simulink model "Final"  (R2018b)
settings: Solver=FixedStepAuto  StartTime=0.0  StopTime=1  RelTol=1e-3  EnableMultiTasking=on
values from neighbouring files (symbols this model uses):
  A = [-(bm*(n^2) + bg)/(Jm*(n^2) + Jg) Kt*n/(Jm*(n^2) + Jg) ... (first row only)    [DC_motor_geared_integral_discrete_sysid23.m]    (also in DC_motor_geared_lqr_discrete_sysid23.m; finalScript.m; finalScriptV2.m; precompensatorVSintegrator.m)
  B = [0 ... (first row only)    [DC_motor_geared_integral_discrete_sysid23.m]    (also in DC_motor_geared_lqr_discrete_sysid23.m; finalScript.m; finalScriptV2.m; precompensatorVSintegrator.m)
  C = [1 0]    [DC_motor_geared_integral_discrete_sysid23.m]    (also in DC_motor_geared_lqr_discrete_sysid23.m = eye(2); finalScript.m; finalScriptV2.m; precompensatorVSintegrator.m = eye(2))
  D = [0]    [DC_motor_geared_integral_discrete_sysid23.m]    (also in DC_motor_geared_lqr_discrete_sysid23.m = [0;0]; finalScript.m; finalScriptV2.m; precompensatorVSintegrator.m)
  Kdi = dlqr(Ad,Bd,Q,R)    [finalScript.m]    (also in finalScriptV2.m)
  n = 16.5    [DC_motor_geared_integral_discrete_sysid23.m]    (also in DC_motor_geared_lqr_discrete_sysid23.m; finalScript.m; finalScriptV2.m)
  Tsc = 1/20000    (= 5e-05)    [DC_motor_geared_integral_discrete_sysid23.m]    (also in DC_motor_geared_lqr_discrete_sysid23.m = 1e-05; finalScript.m; finalScriptV2.m = 0.001)
undefined symbols (not defined in the file or in its folder): DiscIntNeverNeededParam
libraries: dspswit3 x29, simulink x10, powerlib_meascontrol x4, dspsigops x4, pePwmGenerator x4, peLuenbergerObserver x2, peGeneralControl x1
settings Model: Creator=Roberto  LastModifiedBy=Roberto
settings SolverCC: AutoInsertRateTranBlk=on
settings OptimizationCC: EnhancedBackFolding=on  PassReuseOutputArgsAs=Individual arguments  MaxStackSize=64  OptimizeBlockOrder=speed  DifferentSizesBufferReuse=on  OptimizationCustomize=off
settings DebuggingCC: ParameterTunabilityLossMsg=error
settings HardwareCC: ProdBitPerPointer=32  ProdBitPerSizeT=32  ProdBitPerPtrDiffT=32  ProdLargestAtomicInteger=Long  ProdLargestAtomicFloat=Double  ProdWordSize=32  ProdHWDeviceType=ARM Compatible->ARM Cortex
settings SFSimCC: MATLABDynamicMemAlloc=off
settings RTWCC: SystemTargetFile=ert.tlc  HardwareBoard=STM32F746G-Discovery  TemplateMakefile=ert_default_tmf  GenerateReport=on  Toolchain=GNU Tools for ARM Embedded Processors  IncludeHyperlinkInReport=on  LaunchReport=on  GenerateTraceInfo=on  GenerateTraceReport=on  GenerateTraceReportSl=on  GenerateTraceReportSf=on  GenerateTraceReportEml=on
settings CodeAppCC: ForceParamTrailComments=on  IgnoreCustomStorageClasses=off  OperatorAnnotations=on  SimulinkDataObjDesc=on  SFDataObjDesc=on  InsertBlockDesc=on

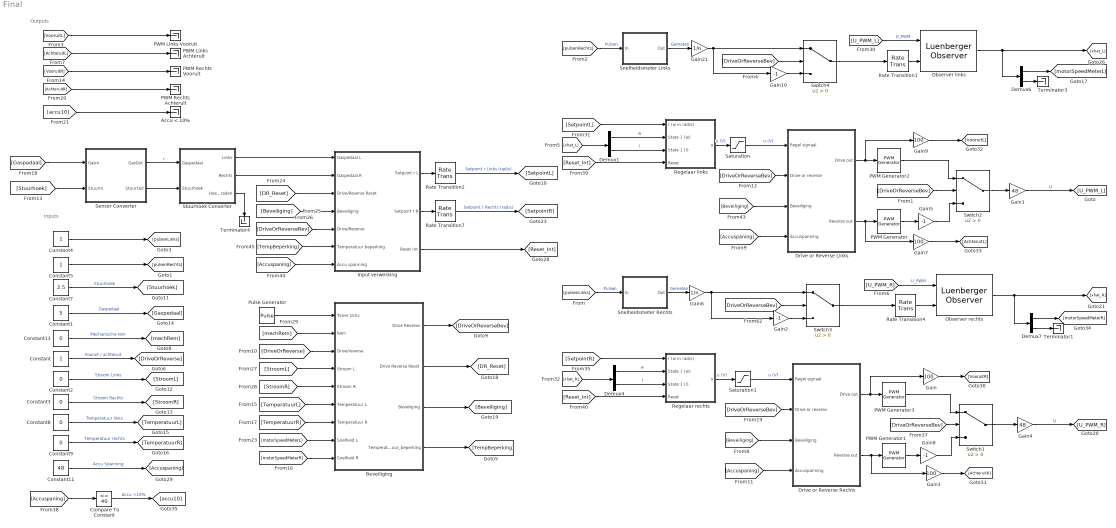
== system Final ==
  note: Inputs
  note: Outputs
  Accu < 10% : Terminator
  Beveiliging : Subsystem
  Compare To Constant : simulink/Logic and Bit Operations/Compare To Constant  relop=<=  const=40  OutDataTypeStr=boolean
  Constant : Constant
  Constant1 : Constant  Value=5
  Constant11 : Constant  Value=48
  Constant{2..3,8..9,13} (5 alike) : Constant  Value=0
  Constant4 : Constant
  Constant5 : Constant
  Constant7 : Constant  Value=2.5
  Demux{1,4,6..7} (4 alike) : Demux  Outputs=2
  Drive or Reverse Links : Subsystem
  Drive or Reverse Rechts : Subsystem
  Gain{,3,7,9} (4 alike) : Gain  Gain=100
  Gain1 : Gain  Gain=48
  Gain{2,5,8,10} (4 alike) : Gain  Gain=-1
  Gain21 : Gain  Gain=1/n
  Gain4 : Gain  Gain=48
  Gain6 : Gain  Gain=1/n
  Input verwerking : Subsystem
  Observer links : peLuenbergerObserver/Luenberger Observer  StateSpaceType=Continuous-time  Ad=Adh  Bd=Bdh  Cd=C  Dd=0  A=A  B=B  C=C  D=D  ObserverDesign=Observer gain  Ld=L  DesiredEigenvalues=eigenVal  x0=[0 0]  Tsd=0.1  Ts=1e-6
  Observer rechts : peLuenbergerObserver/Luenberger Observer  StateSpaceType=Continuous-time  Ad=Adh  Bd=Bdh  Cd=C  Dd=0  A=A  B=B  C=C  D=D  ObserverDesign=Observer gain  Ld=L  DesiredEigenvalues=eigenVal  x0=[0 0]  Tsd=0.1  Ts=1e-6
  PWM Generator{,1..3} (4 alike) : pePwmGenerator/PWM Generator  CarrCount=Up  Tper=1/20000  Ts=1e-6
  PWM Links Achteruit : Terminator
  PWM Links Vooruit : Terminator
  PWM Rechts Achteruit : Terminator
  PWM Rechts Vooruit : Terminator
  Pulse Generator : DiscretePulseGenerator  SampleTime=1/2000
  Rate Transition1 : RateTransition  OutPortSampleTime=1e-6
  Rate Transition2 : RateTransition  OutPortSampleTime=Tsc
  Rate Transition4 : RateTransition  OutPortSampleTime=1e-6
  Rate Transition7 : RateTransition  OutPortSampleTime=Tsc
  Regelaar links : Subsystem
  Regelaar rechts : Subsystem
  Saturation : Saturate  UpperLimit=60  LowerLimit=-60
  Saturation1 : Saturate  UpperLimit=60  LowerLimit=-60
  Sensor Converter : Subsystem
  Snelheidsmeter Links : Subsystem
  Snelheidsmeter Rechts : Subsystem
  Stuurhoek Converter : Subsystem
  Switch{1..4} (4 alike) : Switch  Criteria=u2 > Threshold
  Terminator1 : Terminator
  Terminator3 : Terminator
  Terminator4 : Terminator
  wires:
  Gain1/1 -> [U_PWM_L]  "U"
  Switch2/1 -> Gain1/1
  Demux1/2 -> Regelaar links/3(State 1 (I))  "I"
  Demux1/1 -> Regelaar links/2(State 1 (w))  "w"
  [Reset_Int] -> Regelaar links/4(Reset)
  [xhat_L] -> Demux1/1
  [U_PWM_L] -> Observer links/1  "U_PWM"
  [pulsenRechts] -> Snelheidsmeter Links/1(In)  "Pulsen"
  Rate Transition1/1 -> Observer links/2
  Snelheidsmeter Links/1(Out) -> Gain21/1  "Gemeten"
  Switch4/1 -> Rate Transition1/1
  Observer links/1 -> Demux6/1, [xhat_L]
  Beveiliging/1("Drive Reverse ") -> [DriveOrReverseBev]
  [Gaspedaal] -> Sensor Converter/1(GasIn)
  Stuurhoek Converter/1(Links) -> Input verwerking/1(Gaspedaal L)
  Input verwerking/1(Setpoint r L) -> Rate Transition2/1
  [Stuurhoek] -> Sensor Converter/2(StuurIn)
  Input verwerking/3(Reset Int) -> [Reset_Int]
  Sensor Converter/2(StuurOut) -> Stuurhoek Converter/2(Stuurhoek)
  [DriveOrReverse] -> Beveiliging/3(Drive/reverse)
  [motorSpeedMeterR] -> Beveiliging/9(Snelheid R)
  [TemperatuurL] -> Beveiliging/6(Temperatuur L)
  [StroomR] -> Beveiliging/5(Stroom R)
  [StroomL] -> Beveiliging/4(Stroom L)
  Beveiliging/3(Beveiliging) -> [Beveiliging]
  [motorSpeedMeterL] -> Beveiliging/8(Snelheid L)
  Input verwerking/2(Setpoint r R) -> Rate Transition7/1
  Beveiliging/2(Drive Reverse Reset) -> [DR_Reset]
  Stuurhoek Converter/2(Rechts) -> Input verwerking/2(Gaspedaal R)
  [mechRem] -> Beveiliging/2(Rem)
  [DR_Reset] -> Input verwerking/3(Drive/Reverse Reset)
  [Beveiliging] -> Input verwerking/4(Beveiliging)
  Pulse Generator/1 -> Beveiliging/1(Timer 1khz)
  [DriveOrReverseBev] -> Input verwerking/5(Drive/Reverse)
  Rate Transition7/1 -> [SetpointR]  "Setpoint r Rechts (rad/s)"
  Rate Transition2/1 -> [SetpointL]  "Setpoint r Links (rad/s)"
  [TemperatuurR] -> Beveiliging/7(Temperatuur R)
  Observer rechts/1 -> Demux7/1, [xhat_R]
  Demux4/2 -> Regelaar rechts/3(State 1 (I))  "I"
  Rate Transition4/1 -> Observer rechts/2
  Switch1/1 -> Gain4/1
  [U_PWM_R] -> Observer rechts/1  "U_PWM"
  Snelheidsmeter Rechts/1(Out) -> Gain6/1  "Gemeten"
  [Reset_Int] -> Regelaar rechts/4(Reset)
  [xhat_R] -> Demux4/1
  [pulsenLinks] -> Snelheidsmeter Rechts/1(In)  "Pulsen"
  Demux4/1 -> Regelaar rechts/2(State 1 (w))  "w"
  Gain4/1 -> [U_PWM_R]  "U"
  [SetpointL] -> Regelaar links/1(r (w in rad/s))
  [SetpointR] -> Regelaar rechts/1(r (w in rad/s))
  [Beveiliging] -> Drive or Reverse Rechts/3(Beveiliging)
  [DriveOrReverseBev] -> Switch1/2
  Drive or Reverse Rechts/1(Drive out) -> Gain/1, PWM Generator3/1
  [Accuspaning] -> Drive or Reverse Rechts/4(Accuspanning)
  [DriveOrReverseBev] -> Drive or Reverse Rechts/2(Drive or reverse)
  Drive or Reverse Rechts/2(Reverse out) -> Gain3/1, PWM Generator1/1
  Regelaar rechts/1(u) -> Saturation1/1  "u (V)"
  [Beveiliging] -> Drive or Reverse Links/3(Beveiliging)
  [DriveOrReverseBev] -> Switch2/2
  Drive or Reverse Links/1(Drive out) -> Gain9/1, PWM Generator2/1
  [Accuspaning] -> Drive or Reverse Links/4(Accuspanning)
  [DriveOrReverseBev] -> Drive or Reverse Links/2(Drive or reverse)
  Drive or Reverse Links/2(Reverse out) -> Gain7/1, PWM Generator/1
  Regelaar links/1(u) -> Saturation/1  "u (V)"
  Constant1/1 -> [Gaspedaal]  "Gaspedaal"
  Constant13/1 -> [mechRem]  "Mechanische rem"
  Constant/1 -> [DriveOrReverse]  "Vooruit / achteruit"
  Constant2/1 -> [StroomL]  "Stroom Links"
  Constant9/1 -> [TemperatuurR]  "Temperatuur rechts"
  Constant7/1 -> [Stuurhoek]  "Stuurhoek"
  Constant3/1 -> [StroomR]  "Stroom Rechts"
  Constant8/1 -> [TemperatuurL]  "Temperatuur links"
  Constant11/1 -> [Accuspaning]  "Accu Spanning"
  Beveiliging/4(Temperatuur_beperking) -> [TempBeperking]
  [Accuspaning] -> Input verwerking/7(Accu spanning)
  [TempBeperking] -> Input verwerking/6(Temperatuur beperking)
  Gain6/1 -> Gain2/1, Switch3/1
  [DriveOrReverseBev] -> Switch3/2
  Gain2/1 -> Switch3/3
  Switch3/1 -> Rate Transition4/1
  Gain21/1 -> Gain10/1, Switch4/1
  Gain10/1 -> Switch4/3
  [DriveOrReverseBev] -> Switch4/2
  Gain5/1 -> Switch2/3
  Gain8/1 -> Switch1/3
  PWM Generator/1 -> Gain5/1
  PWM Generator2/1 -> Switch2/1
  PWM Generator1/1 -> Gain8/1
  PWM Generator3/1 -> Switch1/1
  Saturation/1 -> Drive or Reverse Links/1(Regel signaal)  "u (V)"
  Saturation1/1 -> Drive or Reverse Rechts/1(Regel signaal)  "u (V)"
  Demux6/1 -> [motorSpeedMeterL]
  Demux7/1 -> [motorSpeedMeterR]
  Demux7/2 -> Terminator1/1
  Demux6/2 -> Terminator3/1
  Compare To Constant/1 -> [accu10]  "Accu <10%"
  [Accuspaning] -> Compare To Constant/1
  Sensor Converter/1(GasOut) -> Stuurhoek Converter/1("Gaspedaal ")  "r"
  Stuurhoek Converter/3(Hoek in graden) -> Terminator4/1
  Constant4/1 -> [pulsenLinks]
  Constant5/1 -> [pulsenRechts]
  Gain/1 -> [VooruitR]
  Gain3/1 -> [AchteruitR]
  Gain7/1 -> [AchteruitL]
  Gain9/1 -> [VooruitL]
  [VooruitL] -> PWM Links Vooruit/1
  [AchteruitL] -> PWM Links Achteruit/1
  [VooruitR] -> PWM Rechts Vooruit/1
  [AchteruitR] -> PWM Rechts Achteruit/1
  [accu10] -> Accu < 10%/1

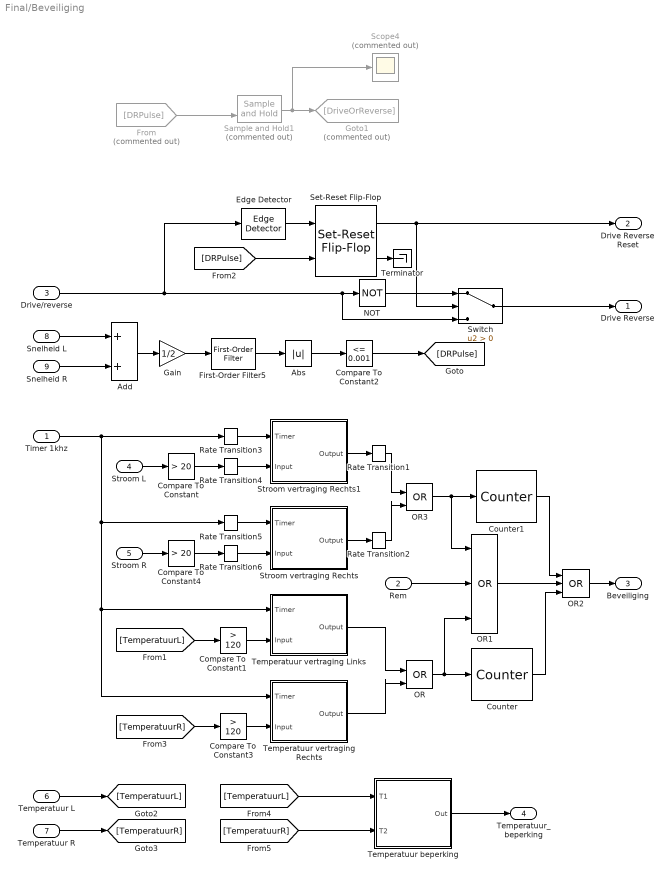
== system Final/Beveiliging ==
  Timer 1khz : Inport
  Rem : Inport  Port=2
  Drive/reverse : Inport  Port=3
  Stroom L : Inport  Port=4
  Stroom R : Inport  Port=5
  Temperatuur L : Inport  Port=6
  Temperatuur R : Inport  Port=7
  Snelheid L : Inport  Port=8
  Snelheid R : Inport  Port=9
  Abs : Abs
  Add : Sum
  Compare To Constant : simulink/Logic and Bit Operations/Compare To Constant  relop=>  const=20  OutDataTypeStr=boolean
  Compare To Constant1 : simulink/Logic and Bit Operations/Compare To Constant  relop=>  const=120  OutDataTypeStr=boolean
  Compare To Constant2 : simulink/Logic and Bit Operations/Compare To Constant  relop=<=  const=0.001  OutDataTypeStr=boolean
  Compare To Constant3 : simulink/Logic and Bit Operations/Compare To Constant  relop=>  const=120  OutDataTypeStr=boolean
  Compare To Constant4 : simulink/Logic and Bit Operations/Compare To Constant  relop=>  const=20  OutDataTypeStr=boolean
  Counter : dspswit3/Counter  Direction=Up  CountEvent=Rising edge  CounterSize=32 bits  MaxCount=255  InitialCount=0  Output=Hit  HitValue=3  ResetInput=off  SamplesPerFrame=1  Ts=1  CntDtype=double  HitDtype=Logical
  Counter1 : dspswit3/Counter  Direction=Up  CountEvent=Rising edge  CounterSize=32 bits  MaxCount=255  InitialCount=0  Output=Hit  HitValue=2  ResetInput=off  SamplesPerFrame=1  Ts=1  CntDtype=double  HitDtype=Logical
  Edge Detector : powerlib_meascontrol/Logic/Edge Detector  model=Either  ic=0  Ts=-1
      settings: SourceProductName=Simscape Power Systems  SourceProductBaseCode=PS
  First-Order Filter5 : powerlib_meascontrol/Filters/First-Order Filter  FilterType=Lowpass  Tc=10e-3  Ts=Tsc  Initialize=on  Vac_Init=[0, 0, 50]  Vdc_Init=0  PlotResponse=off  FreqRange="[0,  200,  1]"
      settings: SourceProductName=Simscape Power Systems
  From : From  Commented=on  GotoTag=DRPulse
  Gain : Gain  Gain=1/2
  Goto1 : Goto  Commented=on  GotoTag=DriveOrReverse
  NOT : Logic  Operator=NOT  IconShape=distinctive  AllPortsSameDT=off  OutDataTypeStr=boolean
  OR : Logic  Operator=OR  IconShape=distinctive  AllPortsSameDT=off  OutDataTypeStr=boolean
  OR1 : Logic  Operator=OR  Inputs=3  IconShape=distinctive  AllPortsSameDT=off  OutDataTypeStr=boolean
  OR2 : Logic  Operator=OR  Inputs=3  IconShape=distinctive  AllPortsSameDT=off  OutDataTypeStr=boolean
  OR3 : Logic  Operator=OR  IconShape=distinctive  AllPortsSameDT=off  OutDataTypeStr=boolean
  Rate Transition{1..6} (6 alike) : RateTransition
  Sample and Hold1 : powerlib_meascontrol/Additional Components/Sample and Hold  Commented=on  ic=0  Ts=0
      settings: SourceProductName=Simscape Power Systems  SourceProductBaseCode=PS
  Scope4 : Scope  Commented=on
  Set-Reset Flip-Flop : peGeneralControl/Set-Reset Flip-Flop  LabelModeActiveChoice=Discrete  UndefState=Set  Q0=0  Ts=-1
  Stroom vertraging Rechts : Subsystem
  Stroom vertraging Rechts1 : Subsystem
  Switch : Switch  Criteria=u2 > Threshold
  Temperatuur beperking : Subsystem
  Temperatuur vertraging Links : Subsystem
  "Temperatuur vertraging Rechts " : Subsystem
  Terminator : Terminator
  "Drive Reverse " : Outport
  Drive Reverse Reset : Outport  Port=2
  Beveiliging : Outport  Port=3
  Temperatuur_beperking : Outport  Port=4
  wires:
  Stroom L/1 -> Compare To Constant/1
  Compare To Constant1/1 -> Temperatuur vertraging Links/2(Input)
  Edge Detector/1 -> Set-Reset Flip-Flop/1
  Set-Reset Flip-Flop/1 -> Switch/2, Drive Reverse Reset/1
  Sample and Hold1/1 -> Scope4/1, Goto1/1
  Abs/1 -> Compare To Constant2/1
  Compare To Constant2/1 -> [DRPulse]
  [DRPulse] -> Set-Reset Flip-Flop/2
  Drive/reverse/1 -> Edge Detector/1, Switch/3, NOT/1
  From/1 -> Sample and Hold1/2
  Snelheid L/1 -> Add/1
  Snelheid R/1 -> Add/2
  Add/1 -> Gain/1
  Gain/1 -> First-Order Filter5/1
  Compare To Constant3/1 -> "Temperatuur vertraging Rechts "/2(Input)
  Timer 1khz/1 -> Rate Transition3/1, Rate Transition5/1, Temperatuur vertraging Links/1(Timer), "Temperatuur vertraging Rechts "/1(Timer)
  Compare To Constant4/1 -> Rate Transition6/1
  Stroom R/1 -> Compare To Constant4/1
  Rem/1 -> OR1/2
  Switch/1 -> "Drive Reverse "/1
  NOT/1 -> Switch/1
  OR/1 -> OR1/3, Counter/1
  Temperatuur vertraging Links/1(Output) -> OR/1
  "Temperatuur vertraging Rechts "/1(Output) -> OR/2
  OR2/1 -> Beveiliging/1
  Counter/1 -> OR2/3
  OR1/1 -> OR2/2
  Set-Reset Flip-Flop/2 -> Terminator/1
  First-Order Filter5/1 -> Abs/1
  Temperatuur L/1 -> [TemperatuurL]
  Temperatuur R/1 -> [TemperatuurR]
  [TemperatuurL] -> Compare To Constant1/1
  [TemperatuurR] -> Compare To Constant3/1
  [TemperatuurL] -> Temperatuur beperking/1(T1)
  [TemperatuurR] -> Temperatuur beperking/2(T2)
  Temperatuur beperking/1(Out) -> Temperatuur_beperking/1
  Compare To Constant/1 -> Rate Transition4/1
  Stroom vertraging Rechts1/1(Output) -> Rate Transition1/1
  Stroom vertraging Rechts/1(Output) -> Rate Transition2/1
  OR3/1 -> Counter1/1, OR1/1
  Counter1/1 -> OR2/1
  Rate Transition6/1 -> Stroom vertraging Rechts/2(Input)
  Rate Transition5/1 -> Stroom vertraging Rechts/1(Timer)
  Rate Transition4/1 -> Stroom vertraging Rechts1/2(Input)
  Rate Transition3/1 -> Stroom vertraging Rechts1/1(Timer)
  Rate Transition2/1 -> OR3/2
  Rate Transition1/1 -> OR3/1

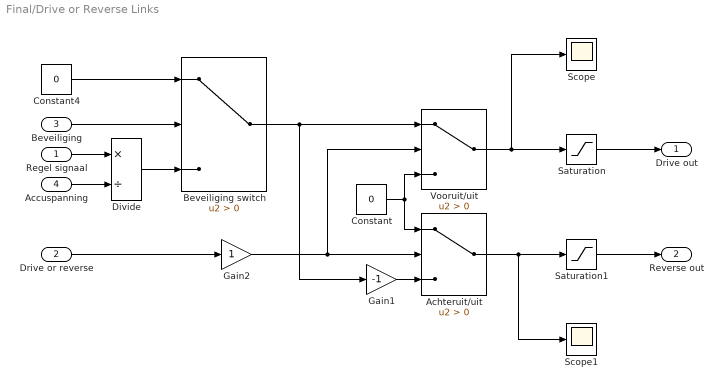
== system Final/Drive or Reverse Links ==
  Regel signaal : Inport
  Drive or reverse : Inport  Port=2
  Beveiliging : Inport  Port=3
  Accuspanning : Inport  Port=4
  Achteruit/uit : Switch  Criteria=u2 > Threshold
  Beveiliging switch : Switch  Criteria=u2 > Threshold
  Constant : Constant  Value=0
  Constant4 : Constant  Value=0
  Divide : Product  Inputs=*/
  Gain1 : Gain  Gain=-1
  Gain2 : Gain
  Saturation : Saturate  UpperLimit=1  LowerLimit=0
  Saturation1 : Saturate  UpperLimit=1  LowerLimit=0
  Scope : Scope
  Scope1 : Scope
  Vooruit/uit : Switch  Criteria=u2 > Threshold
  Drive out : Outport
  Reverse out : Outport  Port=2
  wires:
  Gain1/1 -> Achteruit/uit/3
  Constant4/1 -> Beveiliging switch/1
  Constant/1 -> Achteruit/uit/1, Vooruit/uit/3
  Beveiliging switch/1 -> Gain1/1, Vooruit/uit/1
  Beveiliging/1 -> Beveiliging switch/2
  Achteruit/uit/1 -> Saturation1/1, Scope1/1
  Gain2/1 -> Vooruit/uit/2, Achteruit/uit/2
  Drive or reverse/1 -> Gain2/1
  Vooruit/uit/1 -> Saturation/1, Scope/1
  Accuspanning/1 -> Divide/2
  Divide/1 -> Beveiliging switch/3
  Regel signaal/1 -> Divide/1
  Saturation/1 -> Drive out/1
  Saturation1/1 -> Reverse out/1

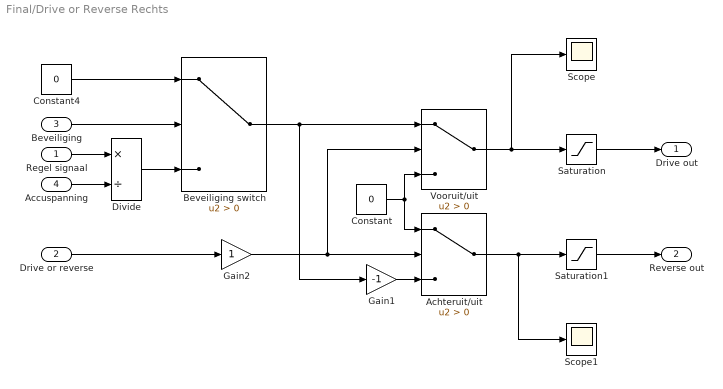
== system Final/Drive or Reverse Rechts ==
  Regel signaal : Inport
  Drive or reverse : Inport  Port=2
  Beveiliging : Inport  Port=3
  Accuspanning : Inport  Port=4
  Achteruit/uit : Switch  Criteria=u2 > Threshold
  Beveiliging switch : Switch  Criteria=u2 > Threshold
  Constant : Constant  Value=0
  Constant4 : Constant  Value=0
  Divide : Product  Inputs=*/
  Gain1 : Gain  Gain=-1
  Gain2 : Gain
  Saturation : Saturate  UpperLimit=1  LowerLimit=0
  Saturation1 : Saturate  UpperLimit=1  LowerLimit=0
  Scope : Scope
  Scope1 : Scope
  Vooruit/uit : Switch  Criteria=u2 > Threshold
  Drive out : Outport
  Reverse out : Outport  Port=2
  wires:
  Gain1/1 -> Achteruit/uit/3
  Constant4/1 -> Beveiliging switch/1
  Constant/1 -> Achteruit/uit/1, Vooruit/uit/3
  Beveiliging switch/1 -> Gain1/1, Vooruit/uit/1
  Beveiliging/1 -> Beveiliging switch/2
  Achteruit/uit/1 -> Saturation1/1, Scope1/1
  Gain2/1 -> Vooruit/uit/2, Achteruit/uit/2
  Drive or reverse/1 -> Gain2/1
  Vooruit/uit/1 -> Saturation/1, Scope/1
  Accuspanning/1 -> Divide/2
  Divide/1 -> Beveiliging switch/3
  Regel signaal/1 -> Divide/1
  Saturation/1 -> Drive out/1
  Saturation1/1 -> Reverse out/1

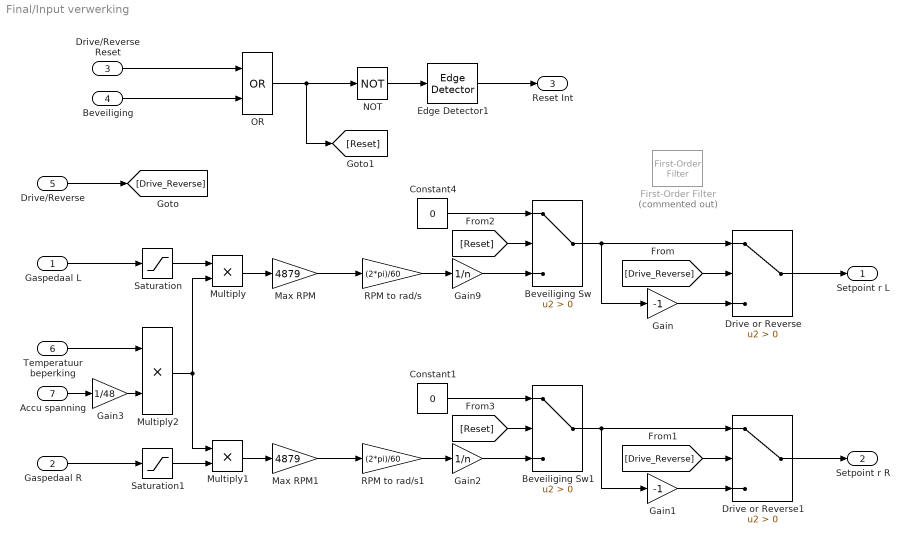
== system Final/Input verwerking ==
  Gaspedaal L : Inport
  Gaspedaal R : Inport  Port=2
  Drive/Reverse Reset : Inport  Port=3
  Beveiliging : Inport  Port=4
  Drive/Reverse : Inport  Port=5
  Temperatuur beperking : Inport  Port=6
  Accu spanning : Inport  Port=7
  Beveiliging Sw : Switch  Criteria=u2 > Threshold
  Beveiliging Sw1 : Switch  Criteria=u2 > Threshold
  Constant1 : Constant  Value=0
  Constant4 : Constant  Value=0
  Drive or Reverse : Switch  Criteria=u2 > Threshold
  Drive or Reverse1 : Switch  Criteria=u2 > Threshold
  Edge Detector1 : dspswit3/Edge Detector  InputProcessing=Columns as channels (frame based)
      settings: SourceProductName=DSP System Toolbox  SourceProductBaseCode=DS
  First-Order Filter : powerlib_meascontrol/Filters/First-Order Filter  Commented=on  FilterType=Lowpass  Tc=10e-2  Ts=0  Initialize=on  Vac_Init=[0, 0, 60]  Vdc_Init=0  PlotResponse=off  FreqRange="[0,  200,  1]"
      settings: SourceProductName=Simscape Power Systems
  Gain : Gain  Gain=-1
  Gain1 : Gain  Gain=-1
  Gain2 : Gain  Gain=1/n
  Gain3 : Gain  Gain=1/48
  Gain9 : Gain  Gain=1/n
  Max RPM : Gain  Gain=4879
  Max RPM1 : Gain  Gain=4879
  Multiply : Product
  Multiply1 : Product
  Multiply2 : Product
  NOT : Logic  Operator=NOT  IconShape=distinctive  AllPortsSameDT=off  OutDataTypeStr=boolean
  OR : Logic  Operator=OR  IconShape=distinctive  AllPortsSameDT=off  OutDataTypeStr=boolean
  RPM to rad/s : Gain  Gain=(2*pi)/60
  RPM to rad/s1 : Gain  Gain=(2*pi)/60
  Saturation : Saturate  UpperLimit=1  LowerLimit=0
  Saturation1 : Saturate  UpperLimit=1  LowerLimit=0
  Setpoint r L : Outport
  Setpoint r R : Outport  Port=2
  Reset Int : Outport  Port=3
  wires:
  Constant4/1 -> Beveiliging Sw/1
  Max RPM/1 -> RPM to rad/s/1
  RPM to rad/s/1 -> Gain9/1
  Gaspedaal L/1 -> Saturation/1
  OR/1 -> [Reset], NOT/1
  Gain9/1 -> Beveiliging Sw/3
  Beveiliging Sw/1 -> Gain/1, Drive or Reverse/1
  Gain/1 -> Drive or Reverse/3
  [Drive_Reverse] -> Drive or Reverse/2
  Drive or Reverse/1 -> Setpoint r L/1
  Edge Detector1/1 -> Reset Int/1
  NOT/1 -> Edge Detector1/1
  Beveiliging/1 -> OR/2
  Drive/Reverse Reset/1 -> OR/1
  Max RPM1/1 -> RPM to rad/s1/1
  RPM to rad/s1/1 -> Gain2/1
  Drive or Reverse1/1 -> Setpoint r R/1
  Gaspedaal R/1 -> Saturation1/1
  Gain1/1 -> Drive or Reverse1/3
  Beveiliging Sw1/1 -> Gain1/1, Drive or Reverse1/1
  Constant1/1 -> Beveiliging Sw1/1
  [Drive_Reverse] -> Drive or Reverse1/2
  Gain2/1 -> Beveiliging Sw1/3
  Drive/Reverse/1 -> [Drive_Reverse]
  [Reset] -> Beveiliging Sw/2
  [Reset] -> Beveiliging Sw1/2
  Multiply/1 -> Max RPM/1
  Multiply1/1 -> Max RPM1/1
  Saturation1/1 -> Multiply1/2
  Saturation/1 -> Multiply/1
  Multiply2/1 -> Multiply/2, Multiply1/1
  Temperatuur beperking/1 -> Multiply2/1
  Accu spanning/1 -> Gain3/1
  Gain3/1 -> Multiply2/2

== system Final/Regelaar links ==
  r (w in rad/s) : Inport
  State 1 (w) : Inport  Port=2
  State 1 (I) : Inport  Port=3
  Reset : Inport  Port=4
  Discrete-Time Integrator2 : DiscreteIntegrator  gainval=1  ExternalReset=rising  SampleTime=Tsc  ICPrevOutput=DiscIntNeverNeededParam  ICPrevScaledInput=DiscIntNeverNeededParam
  Gain1 : Gain  Gain=Kdi(1:2)  Multiplication=Matrix(K*u)
  Gain4 : Gain  Gain=Kdi(3)
  Mux : Mux  Inputs=2
  Sum1 : Sum  Inputs=|+-
  Sum4 : Sum  Inputs=|+-
  u : Outport
  wires:
  r (w in rad/s)/1 -> Sum1/1
  State 1 (I)/1 -> Mux/2
  Mux/1 -> Gain1/1
  Gain1/1 -> Sum4/2
  Gain4/1 -> Sum4/1
  Sum4/1 -> u/1
  State 1 (w)/1 -> Mux/1, Sum1/2
  Sum1/1 -> Discrete-Time Integrator2/1
  Discrete-Time Integrator2/1 -> Gain4/1
  Reset/1 -> Discrete-Time Integrator2/2

== system Final/Regelaar rechts ==
  r (w in rad/s) : Inport
  State 1 (w) : Inport  Port=2
  State 1 (I) : Inport  Port=3
  Reset : Inport  Port=4
  Discrete-Time Integrator2 : DiscreteIntegrator  gainval=1  ExternalReset=rising  SampleTime=Tsc  ICPrevOutput=DiscIntNeverNeededParam  ICPrevScaledInput=DiscIntNeverNeededParam
  Gain1 : Gain  Gain=Kdi(1:2)  Multiplication=Matrix(K*u)
  Gain4 : Gain  Gain=Kdi(3)
  Mux : Mux  Inputs=2
  Sum1 : Sum  Inputs=|+-
  Sum4 : Sum  Inputs=|+-
  u : Outport
  wires:
  r (w in rad/s)/1 -> Sum1/1
  State 1 (I)/1 -> Mux/2
  Mux/1 -> Gain1/1
  Gain1/1 -> Sum4/2
  Gain4/1 -> Sum4/1
  Sum4/1 -> u/1
  State 1 (w)/1 -> Mux/1, Sum1/2
  Sum1/1 -> Discrete-Time Integrator2/1
  Discrete-Time Integrator2/1 -> Gain4/1
  Reset/1 -> Discrete-Time Integrator2/2

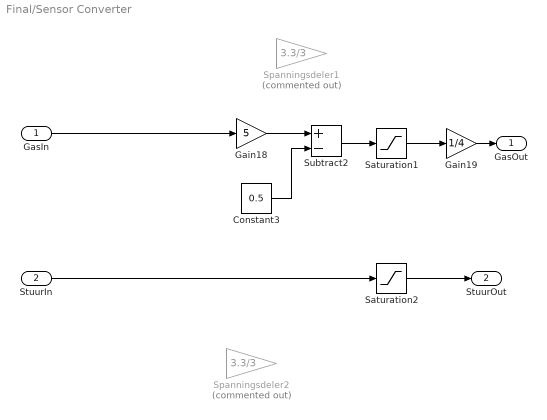
== system Final/Sensor Converter ==
  GasIn : Inport
  StuurIn : Inport  Port=2
  Constant3 : Constant  Value=0.5
  Gain18 : Gain  Gain=5
  Gain19 : Gain  Gain=1/4
  Saturation1 : Saturate  UpperLimit=4  LowerLimit=0
  Saturation2 : Saturate  UpperLimit=1  LowerLimit=0
  Spanningsdeler1 : Gain  Commented=on  Gain=3.3/3
  Spanningsdeler2 : Gain  Commented=on  Gain=3.3/3
  Subtract2 : Sum  Inputs=+-
  GasOut : Outport
  StuurOut : Outport  Port=2
  wires:
  Constant3/1 -> Subtract2/2
  Saturation1/1 -> Gain19/1
  GasIn/1 -> Gain18/1
  Gain18/1 -> Subtract2/1
  Gain19/1 -> GasOut/1
  Subtract2/1 -> Saturation1/1
  Saturation2/1 -> StuurOut/1
  StuurIn/1 -> Saturation2/1

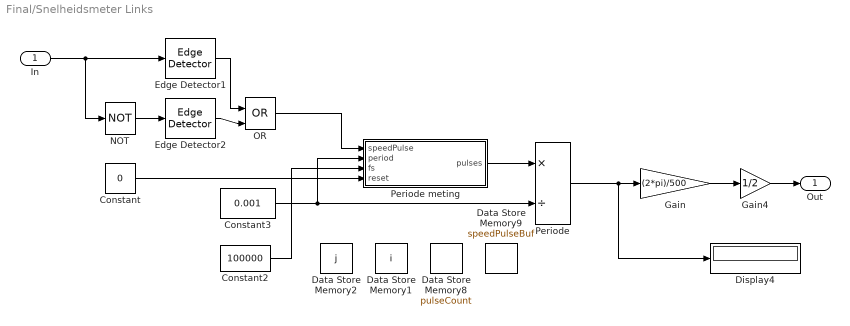
== system Final/Snelheidsmeter Links ==
  In : Inport
  Constant : Constant  Value=0
  Constant2 : Constant  Value=100000
  Constant3 : Constant  Value=0.001
  Data Store Memory1 : DataStoreMemory  DataStoreName=i  ReadBeforeWriteMsg=warning  WriteAfterWriteMsg=warning  WriteAfterReadMsg=warning  InitialValue=1  ShowAdditionalParam=off  OutDataTypeStr=uint32
  Data Store Memory2 : DataStoreMemory  DataStoreName=j  ReadBeforeWriteMsg=warning  WriteAfterWriteMsg=warning  WriteAfterReadMsg=warning  InitialValue=2  ShowAdditionalParam=off  OutDataTypeStr=uint32
  Data Store Memory8 : DataStoreMemory  DataStoreName=pulseCount  ReadBeforeWriteMsg=warning  WriteAfterWriteMsg=warning  WriteAfterReadMsg=warning  ShowAdditionalParam=off  OutDataTypeStr=uint32
  Data Store Memory9 : DataStoreMemory  DataStoreName=speedPulseBuf  ReadBeforeWriteMsg=warning  WriteAfterWriteMsg=warning  WriteAfterReadMsg=warning  ShowAdditionalParam=off  OutDataTypeStr=uint8  Dimensions=10001
  Display4 : Display
  Edge Detector1 : dspswit3/Edge Detector  InputProcessing=Columns as channels (frame based)
      settings: SourceProductName=DSP System Toolbox  SourceProductBaseCode=DS
  Edge Detector2 : dspswit3/Edge Detector  InputProcessing=Columns as channels (frame based)
      settings: SourceProductName=DSP System Toolbox  SourceProductBaseCode=DS
  Gain : Gain  Gain=(2*pi)/500
  Gain4 : Gain  Gain=1/2
  NOT : Logic  Operator=NOT  IconShape=distinctive  AllPortsSameDT=off  OutDataTypeStr=boolean
  OR : Logic  Operator=OR  IconShape=distinctive  AllPortsSameDT=off  OutDataTypeStr=boolean
  Periode : Product  Inputs=*/
  Periode meting : MATLAB Function  TreatAsAtomicUnit=on
  Out : Outport
  wires:
  Constant3/1 -> Periode/2, Periode meting/2(period)
  Periode/1 -> Gain/1, Display4/1
  Constant2/1 -> Periode meting/3(fs)
  Periode meting/1(pulses) -> Periode/1
  In/1 -> NOT/1, Edge Detector1/1
  Gain/1 -> Gain4/1
  Constant/1 -> Periode meting/4(reset)
  OR/1 -> Periode meting/1(speedPulse)
  Edge Detector1/1 -> OR/1
  Edge Detector2/1 -> OR/2
  NOT/1 -> Edge Detector2/1
  Gain4/1 -> Out/1

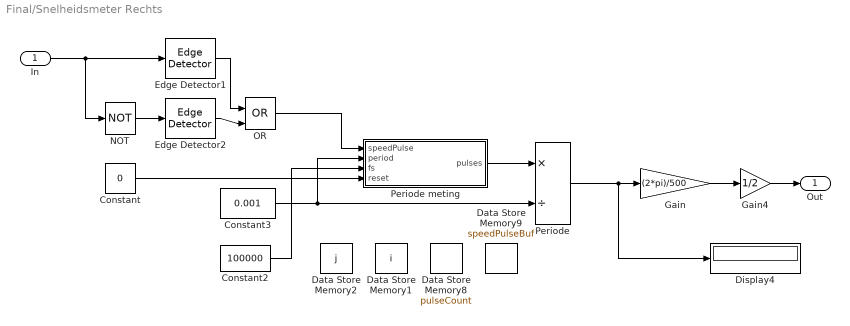
== system Final/Snelheidsmeter Rechts ==
  In : Inport
  Constant : Constant  Value=0
  Constant2 : Constant  Value=100000
  Constant3 : Constant  Value=0.001
  Data Store Memory1 : DataStoreMemory  DataStoreName=i  ReadBeforeWriteMsg=warning  WriteAfterWriteMsg=warning  WriteAfterReadMsg=warning  InitialValue=1  ShowAdditionalParam=off  OutDataTypeStr=uint32
  Data Store Memory2 : DataStoreMemory  DataStoreName=j  ReadBeforeWriteMsg=warning  WriteAfterWriteMsg=warning  WriteAfterReadMsg=warning  InitialValue=2  ShowAdditionalParam=off  OutDataTypeStr=uint32
  Data Store Memory8 : DataStoreMemory  DataStoreName=pulseCount  ReadBeforeWriteMsg=warning  WriteAfterWriteMsg=warning  WriteAfterReadMsg=warning  ShowAdditionalParam=off  OutDataTypeStr=uint32
  Data Store Memory9 : DataStoreMemory  DataStoreName=speedPulseBuf  ReadBeforeWriteMsg=warning  WriteAfterWriteMsg=warning  WriteAfterReadMsg=warning  ShowAdditionalParam=off  OutDataTypeStr=uint8  Dimensions=10001
  Display4 : Display
  Edge Detector1 : dspswit3/Edge Detector  InputProcessing=Columns as channels (frame based)
      settings: SourceProductName=DSP System Toolbox  SourceProductBaseCode=DS
  Edge Detector2 : dspswit3/Edge Detector  InputProcessing=Columns as channels (frame based)
      settings: SourceProductName=DSP System Toolbox  SourceProductBaseCode=DS
  Gain : Gain  Gain=(2*pi)/500
  Gain4 : Gain  Gain=1/2
  NOT : Logic  Operator=NOT  IconShape=distinctive  AllPortsSameDT=off  OutDataTypeStr=boolean
  OR : Logic  Operator=OR  IconShape=distinctive  AllPortsSameDT=off  OutDataTypeStr=boolean
  Periode : Product  Inputs=*/
  Periode meting : MATLAB Function  TreatAsAtomicUnit=on
  Out : Outport
  wires:
  Constant3/1 -> Periode/2, Periode meting/2(period)
  Periode/1 -> Gain/1, Display4/1
  Constant2/1 -> Periode meting/3(fs)
  Periode meting/1(pulses) -> Periode/1
  In/1 -> NOT/1, Edge Detector1/1
  Gain/1 -> Gain4/1
  Constant/1 -> Periode meting/4(reset)
  OR/1 -> Periode meting/1(speedPulse)
  Edge Detector1/1 -> OR/1
  Edge Detector2/1 -> OR/2
  NOT/1 -> Edge Detector2/1
  Gain4/1 -> Out/1

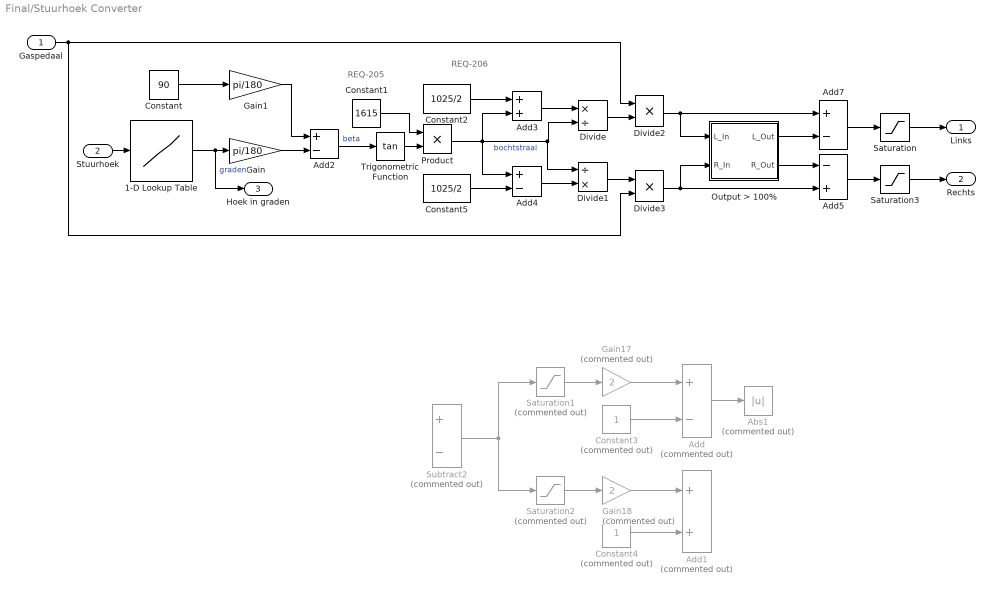
== system Final/Stuurhoek Converter ==
  note: REQ-205
  note: REQ-206
  "Gaspedaal " : Inport
  Stuurhoek : Inport  Port=2
  1-D Lookup Table : Lookup_n-D  NumberOfTableDimensions=1  BreakpointsForDimension1=[0 0.5 1]  Table=[-30 0 30]  InternalRulePriority=Speed  RndMeth=Simplest  InputSameDT=on
  Abs1 : Abs  Commented=on
  Add : Sum  Commented=on  Inputs=+-
  Add1 : Sum  Commented=on
  Add2 : Sum  Inputs=+-
  Add3 : Sum
  Add4 : Sum  Inputs=+-
  Add5 : Sum  Inputs=-+
  Add7 : Sum  Inputs=+-
  Constant : Constant  Value=90
  Constant1 : Constant  Value=1615
  Constant2 : Constant  Value=1025/2
  Constant3 : Constant  Commented=on
  Constant4 : Constant  Commented=on
  Constant5 : Constant  Value=1025/2
  Divide : Product  Inputs=*/
  Divide1 : Product  Inputs=/*
  Divide2 : Product  Inputs=**
  Divide3 : Product  Inputs=**
  Gain : Gain  Gain=pi/180
  Gain1 : Gain  Gain=pi/180
  Gain17 : Gain  Commented=on  Gain=2
  Gain18 : Gain  Commented=on  Gain=2
  Output > 100% : Subsystem
  Product : Product
  Saturation : Saturate  UpperLimit=1  LowerLimit=0
  Saturation1 : Saturate  Commented=on  LowerLimit=0
  Saturation2 : Saturate  Commented=on  UpperLimit=0
  Saturation3 : Saturate  UpperLimit=1  LowerLimit=0
  Subtract2 : Sum  Commented=on  Inputs=+-
  Trigonometric Function : Trigonometry  Operator=tan
  Links : Outport
  Rechts : Outport  Port=2
  Hoek in graden : Outport  Port=3
  wires:
  Saturation1/1 -> Gain17/1
  Subtract2/1 -> Saturation2/1, Saturation1/1
  Gain18/1 -> Add1/1
  Add/1 -> Abs1/1
  Saturation2/1 -> Gain18/1
  Gain17/1 -> Add/1
  Constant4/1 -> Add1/2
  Constant3/1 -> Add/2
  1-D Lookup Table/1 -> Hoek in graden/1, Gain/1  "graden"
  Constant/1 -> Gain1/1
  Add2/1 -> Trigonometric Function/1  "beta"
  Constant1/1 -> Product/1
  Trigonometric Function/1 -> Product/2
  Product/1 -> Divide1/1, Divide/2, Add4/1, Add3/2  "bochtstraal"
  Constant2/1 -> Add3/1
  Add3/1 -> Divide/1
  Constant5/1 -> Add4/2
  Add4/1 -> Divide1/2
  Divide1/1 -> Divide3/1
  Divide/1 -> Divide2/2
  "Gaspedaal "/1 -> Divide2/1, Divide3/2
  Divide2/1 -> Add7/1, Output > 100%/1(L_In)
  Divide3/1 -> Output > 100%/2(R_In), Add5/2
  Stuurhoek/1 -> 1-D Lookup Table/1
  Gain/1 -> Add2/2
  Gain1/1 -> Add2/1
  Add7/1 -> Saturation/1
  Add5/1 -> Saturation3/1
  Output > 100%/1(L_Out) -> Add7/2
  Output > 100%/2(R_Out) -> Add5/1
  Saturation/1 -> Links/1
  Saturation3/1 -> Rechts/1

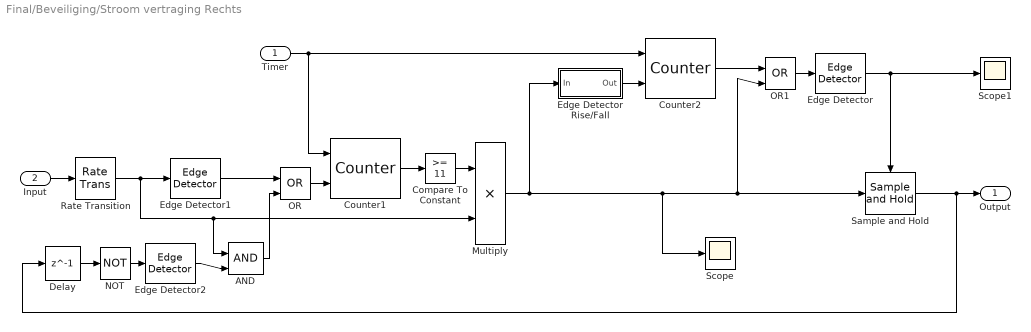
== system Final/Beveiliging/Stroom vertraging Rechts ==
  Timer : Inport
  Input : Inport  Port=2
  AND : Logic  IconShape=distinctive  AllPortsSameDT=off  OutDataTypeStr=boolean
  Compare To Constant : simulink/Logic and Bit Operations/Compare To Constant  relop=>=  const=11  OutDataTypeStr=boolean
  Counter1 : dspswit3/Counter  Direction=Up  CountEvent=Rising edge  CounterSize=32 bits  MaxCount=20  InitialCount=0  Output=Count  HitValue=20  ResetInput=on  SamplesPerFrame=1  Ts=1  CntDtype=double  HitDtype=Logical
  Counter2 : dspswit3/Counter  Direction=Up  CountEvent=Rising edge  CounterSize=User defined  MaxCount=201  InitialCount=0  Output=Hit  HitValue=201  ResetInput=on  SamplesPerFrame=1  Ts=1  CntDtype=double  HitDtype=Logical
  Delay : Delay  DelayLength=1
  Edge Detector : dspswit3/Edge Detector  InputProcessing=Columns as channels (frame based)
      settings: SourceProductName=DSP System Toolbox  SourceProductBaseCode=DS
  Edge Detector1 : dspswit3/Edge Detector  InputProcessing=Columns as channels (frame based)
      settings: SourceProductName=DSP System Toolbox  SourceProductBaseCode=DS
  Edge Detector2 : dspswit3/Edge Detector  InputProcessing=Columns as channels (frame based)
      settings: SourceProductName=DSP System Toolbox  SourceProductBaseCode=DS
  Edge Detector Rise/Fall : Subsystem
  Multiply : Product
  NOT : Logic  Operator=NOT  IconShape=distinctive  AllPortsSameDT=off  OutDataTypeStr=boolean
  OR : Logic  Operator=OR  IconShape=distinctive  AllPortsSameDT=off  OutDataTypeStr=boolean
  OR1 : Logic  Operator=OR  IconShape=distinctive  AllPortsSameDT=off  OutDataTypeStr=boolean
  Rate Transition : RateTransition  OutPortSampleTime=1/1000
  Sample and Hold : dspsigops/Sample and Hold  trig=Rising edge  initCond=0  latchinput=off
  Scope : Scope
  Scope1 : Scope
  Output : Outport
  wires:
  Timer/1 -> Counter2/1, Counter1/1
  Sample and Hold/1 -> Output/1, Delay/1
  OR1/1 -> Edge Detector/1
  Edge Detector/1 -> Scope1/1, Sample and Hold/Trigger
  Counter2/1 -> OR1/1
  Multiply/1 -> Edge Detector Rise/Fall/1(In), OR1/2, Sample and Hold/1, Scope/1
  Edge Detector Rise/Fall/1(Out) -> Counter2/2
  Counter1/1 -> Compare To Constant/1
  Input/1 -> Rate Transition/1
  Rate Transition/1 -> Multiply/2, AND/1, Edge Detector1/1
  NOT/1 -> Edge Detector2/1
  Edge Detector2/1 -> AND/2
  AND/1 -> OR/2
  OR/1 -> Counter1/2
  Edge Detector1/1 -> OR/1
  Delay/1 -> NOT/1
  Compare To Constant/1 -> Multiply/1

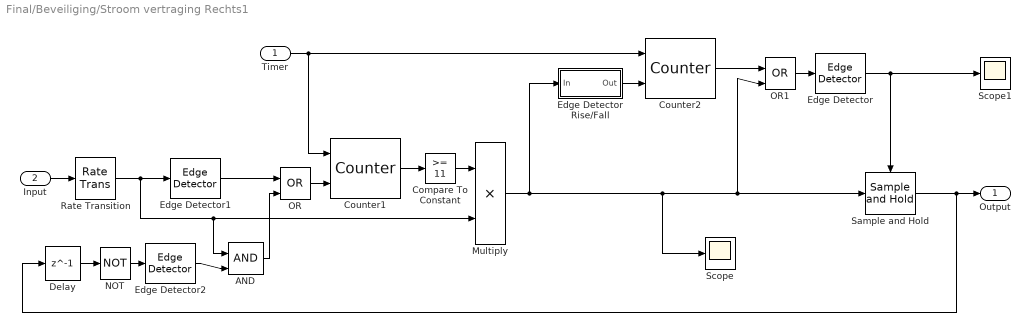
== system Final/Beveiliging/Stroom vertraging Rechts1 ==
  Timer : Inport
  Input : Inport  Port=2
  AND : Logic  IconShape=distinctive  AllPortsSameDT=off  OutDataTypeStr=boolean
  Compare To Constant : simulink/Logic and Bit Operations/Compare To Constant  relop=>=  const=11  OutDataTypeStr=boolean
  Counter1 : dspswit3/Counter  Direction=Up  CountEvent=Rising edge  CounterSize=32 bits  MaxCount=20  InitialCount=0  Output=Count  HitValue=20  ResetInput=on  SamplesPerFrame=1  Ts=1  CntDtype=double  HitDtype=Logical
  Counter2 : dspswit3/Counter  Direction=Up  CountEvent=Rising edge  CounterSize=User defined  MaxCount=201  InitialCount=0  Output=Hit  HitValue=201  ResetInput=on  SamplesPerFrame=1  Ts=1  CntDtype=double  HitDtype=Logical
  Delay : Delay  DelayLength=1
  Edge Detector : dspswit3/Edge Detector  InputProcessing=Columns as channels (frame based)
      settings: SourceProductName=DSP System Toolbox  SourceProductBaseCode=DS
  Edge Detector1 : dspswit3/Edge Detector  InputProcessing=Columns as channels (frame based)
      settings: SourceProductName=DSP System Toolbox  SourceProductBaseCode=DS
  Edge Detector2 : dspswit3/Edge Detector  InputProcessing=Columns as channels (frame based)
      settings: SourceProductName=DSP System Toolbox  SourceProductBaseCode=DS
  Edge Detector Rise/Fall : Subsystem
  Multiply : Product
  NOT : Logic  Operator=NOT  IconShape=distinctive  AllPortsSameDT=off  OutDataTypeStr=boolean
  OR : Logic  Operator=OR  IconShape=distinctive  AllPortsSameDT=off  OutDataTypeStr=boolean
  OR1 : Logic  Operator=OR  IconShape=distinctive  AllPortsSameDT=off  OutDataTypeStr=boolean
  Rate Transition : RateTransition  OutPortSampleTime=1/1000
  Sample and Hold : dspsigops/Sample and Hold  trig=Rising edge  initCond=0  latchinput=off
  Scope : Scope
  Scope1 : Scope
  Output : Outport
  wires:
  Timer/1 -> Counter2/1, Counter1/1
  Sample and Hold/1 -> Output/1, Delay/1
  OR1/1 -> Edge Detector/1
  Edge Detector/1 -> Scope1/1, Sample and Hold/Trigger
  Counter2/1 -> OR1/1
  Multiply/1 -> Edge Detector Rise/Fall/1(In), OR1/2, Sample and Hold/1, Scope/1
  Edge Detector Rise/Fall/1(Out) -> Counter2/2
  Counter1/1 -> Compare To Constant/1
  Input/1 -> Rate Transition/1
  Rate Transition/1 -> Multiply/2, AND/1, Edge Detector1/1
  NOT/1 -> Edge Detector2/1
  Edge Detector2/1 -> AND/2
  AND/1 -> OR/2
  OR/1 -> Counter1/2
  Edge Detector1/1 -> OR/1
  Delay/1 -> NOT/1
  Compare To Constant/1 -> Multiply/1

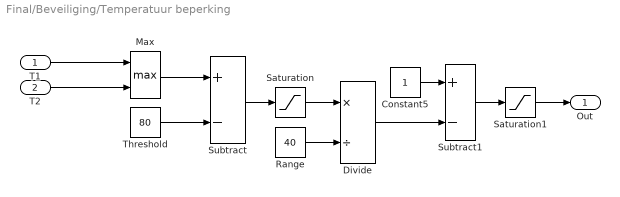
== system Final/Beveiliging/Temperatuur beperking ==
  T1 : Inport
  T2 : Inport  Port=2
  Constant5 : Constant
  Divide : Product  Inputs=*/
  Max : MinMax  Function=max  Inputs=2
  Range : Constant  Value=40
  Saturation : Saturate  UpperLimit=inf  LowerLimit=0
  Saturation1 : Saturate  UpperLimit=1  LowerLimit=0
  Subtract : Sum  Inputs=+-
  Subtract1 : Sum  Inputs=+-
  Threshold : Constant  Value=80
  Out : Outport
  wires:
  Subtract/1 -> Saturation/1
  Divide/1 -> Subtract1/2
  Constant5/1 -> Subtract1/1
  Threshold/1 -> Subtract/2
  Max/1 -> Subtract/1
  T2/1 -> Max/2
  Range/1 -> Divide/2
  Saturation/1 -> Divide/1
  Subtract1/1 -> Saturation1/1
  T1/1 -> Max/1
  Saturation1/1 -> Out/1

== system Final/Beveiliging/Temperatuur vertraging Links ==
  Timer : Inport
  Input : Inport  Port=2
  Counter2 : dspswit3/Counter  Direction=Up  CountEvent=Rising edge  CounterSize=User defined  MaxCount=300  InitialCount=0  Output=Hit  HitValue=300  ResetInput=on  SamplesPerFrame=1  Ts=1  CntDtype=double  HitDtype=Logical
  Edge Detector : dspswit3/Edge Detector  InputProcessing=Columns as channels (frame based)
      settings: SourceProductName=DSP System Toolbox  SourceProductBaseCode=DS
  Edge Detector Rise/Fall : Subsystem
  OR1 : Logic  Operator=OR  IconShape=distinctive  AllPortsSameDT=off  OutDataTypeStr=boolean
  Sample and Hold : dspsigops/Sample and Hold  trig=Rising edge  initCond=0  latchinput=off
  Scope : Scope
  Scope1 : Scope
  Output : Outport
  wires:
  Timer/1 -> Counter2/1
  Sample and Hold/1 -> Output/1
  OR1/1 -> Edge Detector/1
  Edge Detector/1 -> Scope1/1, Sample and Hold/Trigger
  Counter2/1 -> OR1/1
  Input/1 -> Scope/1, OR1/2, Sample and Hold/1, Edge Detector Rise/Fall/1(In)
  Edge Detector Rise/Fall/1(Out) -> Counter2/2

== system Final/Beveiliging/Temperatuur vertraging Rechts  ==
  Timer : Inport
  Input : Inport  Port=2
  Counter2 : dspswit3/Counter  Direction=Up  CountEvent=Rising edge  CounterSize=User defined  MaxCount=300  InitialCount=0  Output=Hit  HitValue=300  ResetInput=on  SamplesPerFrame=1  Ts=1  CntDtype=double  HitDtype=Logical
  Edge Detector : dspswit3/Edge Detector  InputProcessing=Columns as channels (frame based)
      settings: SourceProductName=DSP System Toolbox  SourceProductBaseCode=DS
  Edge Detector Rise/Fall : Subsystem
  OR1 : Logic  Operator=OR  IconShape=distinctive  AllPortsSameDT=off  OutDataTypeStr=boolean
  Sample and Hold : dspsigops/Sample and Hold  trig=Rising edge  initCond=0  latchinput=off
  Scope : Scope
  Scope1 : Scope
  Output : Outport
  wires:
  Timer/1 -> Counter2/1
  Sample and Hold/1 -> Output/1
  OR1/1 -> Edge Detector/1
  Edge Detector/1 -> Scope1/1, Sample and Hold/Trigger
  Counter2/1 -> OR1/1
  Input/1 -> Scope/1, OR1/2, Sample and Hold/1, Edge Detector Rise/Fall/1(In)
  Edge Detector Rise/Fall/1(Out) -> Counter2/2

== system Final/Stuurhoek Converter/Output > 100% ==
  L_In : Inport
  R_In : Inport  Port=2
  Compare To Constant : simulink/Logic and Bit Operations/Compare To Constant  relop=>  const=1  OutDataTypeStr=boolean
  Compare To Constant1 : simulink/Logic and Bit Operations/Compare To Constant  relop=>  const=1  OutDataTypeStr=boolean
  Divide4 : Product  Inputs=**
  Divide5 : Product  Inputs=**
  Subtract : Sum  Inputs=+-
  Subtract1 : Sum  Inputs=-+
  L_Out : Outport
  R_Out : Outport  Port=2
  wires:
  Compare To Constant1/1 -> Subtract1/1, Divide4/1
  Compare To Constant/1 -> Subtract/2, Divide5/2
  Subtract1/1 -> Divide4/2
  Subtract/1 -> Divide5/1
  L_In/1 -> Subtract/1, Compare To Constant/1
  Divide5/1 -> R_Out/1
  R_In/1 -> Subtract1/2, Compare To Constant1/1
  Divide4/1 -> L_Out/1

== system Final/Beveiliging/Stroom vertraging Rechts/Edge Detector Rise//Fall ==
  In : Inport
  Edge Detector1 : dspswit3/Edge Detector  InputProcessing=Columns as channels (frame based)
      settings: SourceProductName=DSP System Toolbox  SourceProductBaseCode=DS
  Edge Detector2 : dspswit3/Edge Detector  InputProcessing=Columns as channels (frame based)
      settings: SourceProductName=DSP System Toolbox  SourceProductBaseCode=DS
  NOT : Logic  Operator=NOT  IconShape=distinctive  AllPortsSameDT=off  OutDataTypeStr=boolean
  OR : Logic  Operator=OR  IconShape=distinctive  AllPortsSameDT=off  OutDataTypeStr=boolean
  Out : Outport
  wires:
  In/1 -> NOT/1, Edge Detector1/1
  NOT/1 -> Edge Detector2/1
  Edge Detector1/1 -> OR/1
  OR/1 -> Out/1
  Edge Detector2/1 -> OR/2

== system Final/Beveiliging/Stroom vertraging Rechts1/Edge Detector Rise//Fall ==
  In : Inport
  Edge Detector1 : dspswit3/Edge Detector  InputProcessing=Columns as channels (frame based)
      settings: SourceProductName=DSP System Toolbox  SourceProductBaseCode=DS
  Edge Detector2 : dspswit3/Edge Detector  InputProcessing=Columns as channels (frame based)
      settings: SourceProductName=DSP System Toolbox  SourceProductBaseCode=DS
  NOT : Logic  Operator=NOT  IconShape=distinctive  AllPortsSameDT=off  OutDataTypeStr=boolean
  OR : Logic  Operator=OR  IconShape=distinctive  AllPortsSameDT=off  OutDataTypeStr=boolean
  Out : Outport
  wires:
  In/1 -> NOT/1, Edge Detector1/1
  NOT/1 -> Edge Detector2/1
  Edge Detector1/1 -> OR/1
  OR/1 -> Out/1
  Edge Detector2/1 -> OR/2

== system Final/Beveiliging/Temperatuur vertraging Links/Edge Detector Rise//Fall ==
  In : Inport
  Edge Detector1 : dspswit3/Edge Detector  InputProcessing=Columns as channels (frame based)
      settings: SourceProductName=DSP System Toolbox  SourceProductBaseCode=DS
  Edge Detector2 : dspswit3/Edge Detector  InputProcessing=Columns as channels (frame based)
      settings: SourceProductName=DSP System Toolbox  SourceProductBaseCode=DS
  NOT : Logic  Operator=NOT  IconShape=distinctive  AllPortsSameDT=off  OutDataTypeStr=boolean
  OR : Logic  Operator=OR  IconShape=distinctive  AllPortsSameDT=off  OutDataTypeStr=boolean
  Out : Outport
  wires:
  In/1 -> NOT/1, Edge Detector1/1
  NOT/1 -> Edge Detector2/1
  Edge Detector1/1 -> OR/1
  OR/1 -> Out/1
  Edge Detector2/1 -> OR/2

== system Final/Beveiliging/Temperatuur vertraging Rechts /Edge Detector Rise//Fall ==
  In : Inport
  Edge Detector1 : dspswit3/Edge Detector  InputProcessing=Columns as channels (frame based)
      settings: SourceProductName=DSP System Toolbox  SourceProductBaseCode=DS
  Edge Detector2 : dspswit3/Edge Detector  InputProcessing=Columns as channels (frame based)
      settings: SourceProductName=DSP System Toolbox  SourceProductBaseCode=DS
  NOT : Logic  Operator=NOT  IconShape=distinctive  AllPortsSameDT=off  OutDataTypeStr=boolean
  OR : Logic  Operator=OR  IconShape=distinctive  AllPortsSameDT=off  OutDataTypeStr=boolean
  Out : Outport
  wires:
  In/1 -> NOT/1, Edge Detector1/1
  NOT/1 -> Edge Detector2/1
  Edge Detector1/1 -> OR/1
  OR/1 -> Out/1
  Edge Detector2/1 -> OR/2

== matlab function Final/Snelheidsmeter Links/Periode meting ==
  data: speedPulse input; pulses output; speedPulseBuf data_store_memory; pulseCount data_store_memory; period input; i data_store_memory; fs input; j data_store_memory; reset input
function pulses = fcn(speedPulse,period, fs, reset)

global pulseCount;
global speedPulseBuf;
global i;
global j;

if reset == 1
    speedPulseBuf = uint8(zeros(size(speedPulseBuf)));
end

bufTime = period*fs + 1;

if i > bufTime
    i = uint32(1);
end

if j > bufTime
    j = uint32(1);
end

speedPulseBuf(i) = speedPulse;
pulseCount = pulseCount + uint32(speedPulse);
pulseCount = pulseCount - uint32(speedPulseBuf(j));

i = i + 1;
j = j + 1;

pulses = pulseCount;

== matlab function Final/Snelheidsmeter Rechts/Periode meting ==
  data: speedPulse input; pulses output; speedPulseBuf data_store_memory; pulseCount data_store_memory; period input; i data_store_memory; fs input; j data_store_memory; reset input
function pulses = fcn(speedPulse,period, fs, reset)

global pulseCount;
global speedPulseBuf;
global i;
global j;

if reset == 1
    speedPulseBuf = uint8(zeros(size(speedPulseBuf)));
end

bufTime = period*fs + 1;

if i > bufTime
    i = uint32(1);
end

if j > bufTime
    j = uint32(1);
end

speedPulseBuf(i) = speedPulse;
pulseCount = pulseCount + uint32(speedPulse);
pulseCount = pulseCount - uint32(speedPulseBuf(j));

i = i + 1;
j = j + 1;

pulses = pulseCount;
